simulink model "Utkarsh_2005574_R_W1_P5"  (R2021a)
settings: Solver=VariableStepAuto  StartTime=0.0  StopTime=10.0  RelTol=1e-3
undefined symbols (not defined in the file): C, R
libraries: simulink x1
settings Model: Creator=Utkarsh Anand  LastModifiedBy=Utkarsh Anand

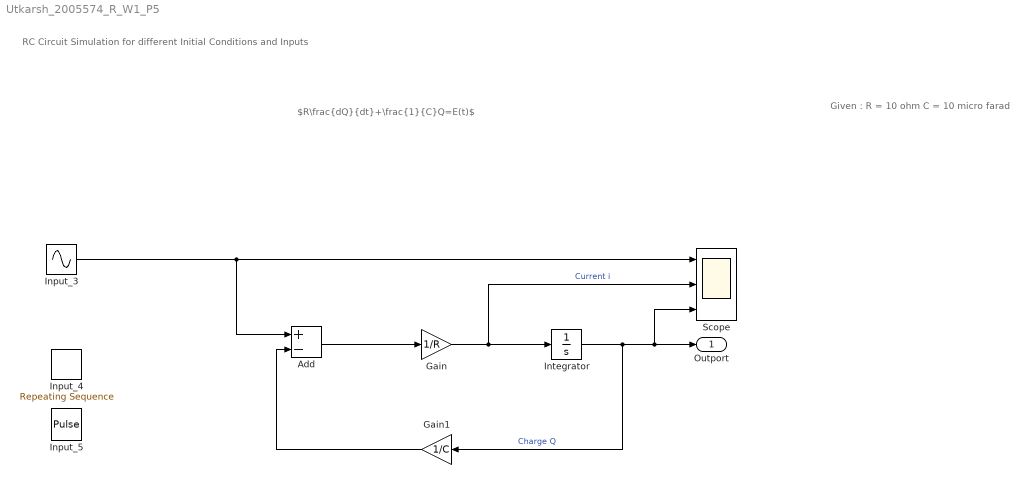
== system Utkarsh_2005574_R_W1_P5 ==
  note: Given :
      | R = 10 ohm
      | C = 10 micro farad
  note: $R\frac{dQ}{dt}+\frac{1}{C}Q=E(t)$
  note: RC Circuit Simulation for different Initial Conditions and Inputs
  Add : Sum  Inputs=+-
  Gain : Gain  Gain=1/R
  Gain1 : Gain  Gain=1/C
  Input_3 : Sin  Frequency=pi  SampleTime=0
  Input_4 : simulink/Sources/Repeating Sequence  rep_seq_t=[0 2]  rep_seq_y=[0 2]
  Input_5 : DiscretePulseGenerator  PulseType=Time based  Period=1  PulseWidth=40
  Integrator : Integrator
  Scope : Scope  NumInputPorts=3
  Outport : Outport
  wires:
  Gain/1 -> Scope/2, Integrator/1  "Current i"
  Integrator/1 -> Gain1/1, Scope/3, Outport/1  "Charge Q"
  Gain1/1 -> Add/2
  Add/1 -> Gain/1
  Input_3/1 -> Add/1, Scope/1
